simulink model "estimator_integrator_syme"  (R2024a)
settings: Solver=VariableStepAuto  StartTime=0.0  StopTime=10.0  RelTol=1e-3
values from neighbouring files (symbols this model uses):
  J = 0.02    [ControlSystemFinal_ChoiChiHyuk.m]
  K_syme = acker(A,B,desired_poles_syme)    [ControlSystemFinal_ChoiChiHyuk.m]
  Kb = 0.015    [ControlSystemFinal_ChoiChiHyuk.m]
  Kf = 0.2    [ControlSystemFinal_ChoiChiHyuk.m]
  Ki_syme = K_aug_syme(end)    [ControlSystemFinal_ChoiChiHyuk.m]
  Km = 0.015    [ControlSystemFinal_ChoiChiHyuk.m]
  Kx_i_syme = K_aug_syme(1:n)    [ControlSystemFinal_ChoiChiHyuk.m]
  L = 0.5    [ControlSystemFinal_ChoiChiHyuk.m]
  L_esti_syme = acker(A,B,desired_error)    [ControlSystemFinal_ChoiChiHyuk.m]
  Nb_syme = Nu + K_syme*Nx    [ControlSystemFinal_ChoiChiHyuk.m]
  R = 2.0    (= 2)    [ControlSystemFinal_ChoiChiHyuk.m]
settings Model: Creator=kevin  LastModifiedBy=kevin

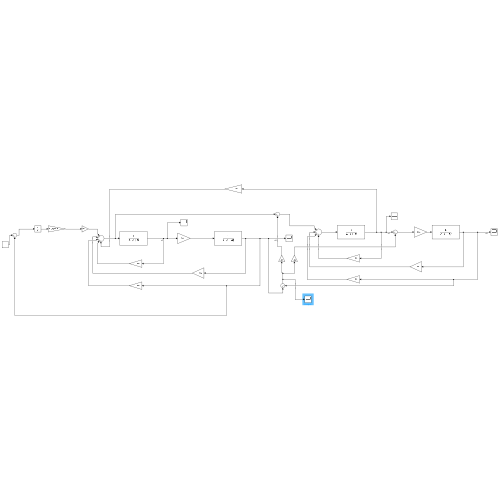
[thumbnail: Simulink's stored preview of the top-level diagram]
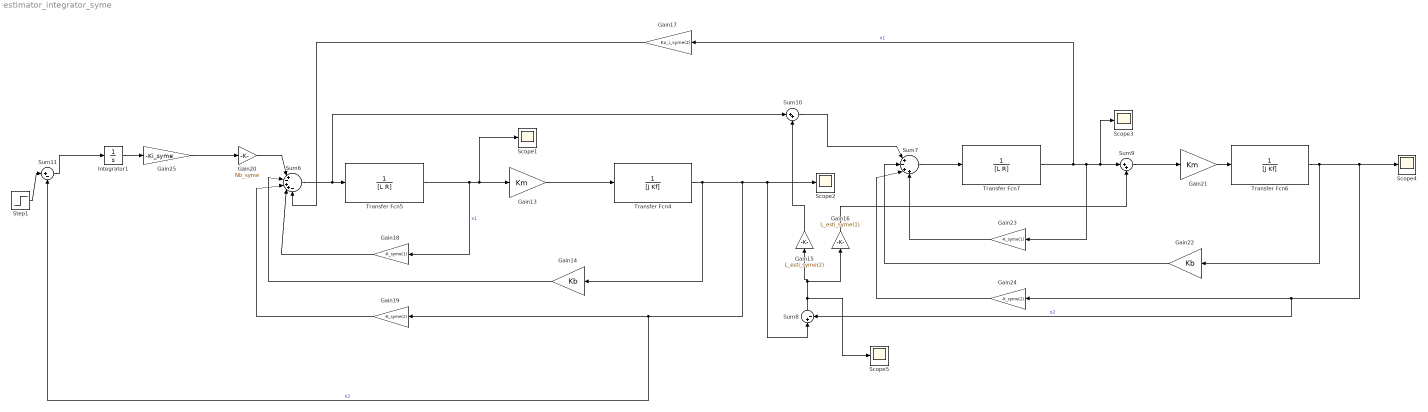
== system estimator_integrator_syme ==
  Gain13 : Gain  Gain=Km
  Gain14 : Gain  Gain=Kb
  Gain15 : Gain  Gain=L_esti_syme(2)
  Gain16 : Gain  Gain=L_esti_syme(1)
  Gain17 : Gain  Gain=Kx_i_syme(2)
  Gain18 : Gain  Gain=-K_syme(1)
  Gain19 : Gain  Gain=-K_syme(2)
  Gain20 : Gain  Gain=Nb_syme
  Gain21 : Gain  Gain=Km
  Gain22 : Gain  Gain=Kb
  Gain23 : Gain  Gain=-K_syme(1)
  Gain24 : Gain  Gain=-K_syme(2)
  Gain25 : Gain  Gain=-Ki_syme
  Integrator1 : Integrator
  Scope{1..5} (5 alike) : Scope
  Step1 : Step  SampleTime=0
  Sum10 : Sum  Inputs=|++
  Sum11 : Sum  Inputs=|+-
  Sum6 : Sum  Inputs=|+-++-
  Sum7 : Sum  Inputs=|+-++
  Sum8 : Sum  Inputs=|+-
  Sum9 : Sum  Inputs=|++
  Transfer Fcn4 : TransferFcn  Denominator=[J Kf]
  Transfer Fcn5 : TransferFcn  Denominator=[L R]
  Transfer Fcn6 : TransferFcn  Denominator=[J Kf]
  Transfer Fcn7 : TransferFcn  Denominator=[L R]
  wires:
  Sum6/1 -> Sum10/1, Transfer Fcn5/1
  Gain19/1 -> Sum6/3
  Sum11/1 -> Integrator1/1
  Transfer Fcn5/1 -> Gain18/1, Scope1/1, Gain13/1  "x1"
  Gain24/1 -> Sum7/3
  Transfer Fcn7/1 -> Gain17/1, Gain23/1, Scope3/1, Sum9/1  "x1"
  Gain14/1 -> Sum6/2
  Gain25/1 -> Gain20/1
  Gain18/1 -> Sum6/4
  Gain20/1 -> Sum6/1
  Sum8/1 -> Scope5/1, Gain16/1, Gain15/1
  Transfer Fcn4/1 -> Sum11/2, Gain19/1, Scope2/1, Sum8/1, Gain14/1  "x2"
  Step1/1 -> Sum11/1
  Sum9/1 -> Gain21/1
  Gain16/1 -> Sum9/2
  Sum7/1 -> Transfer Fcn7/1
  Gain23/1 -> Sum7/4
  Gain13/1 -> Transfer Fcn4/1
  Gain15/1 -> Sum10/2
  Transfer Fcn6/1 -> Scope4/1, Sum8/2, Gain24/1, Gain22/1  "x2"
  Integrator1/1 -> Gain25/1
  Gain22/1 -> Sum7/2
  Gain17/1 -> Sum6/5
  Sum10/1 -> Sum7/1
  Gain21/1 -> Transfer Fcn6/1
